simulink model "State_feedback_controller"  (R2020a)
settings: Solver=VariableStepAuto  StartTime=0.0  StopTime=10.0  RelTol=1e-3
undefined symbols (not defined in the file): Ad, bd, c, d, K1, K2, T
settings Model: Creator=elkin  LastModifiedBy=elkin

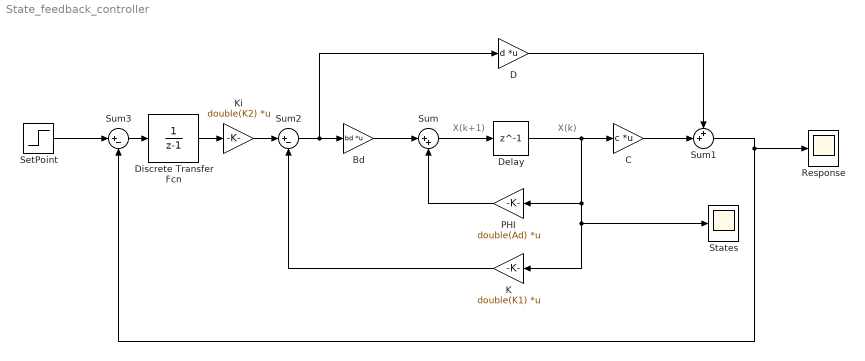
== system State_feedback_controller ==
  note: X(k+1)
  note: X(k)
  Bd : Gain  Gain=bd  Multiplication=Matrix(K*u)
  C : Gain  Gain=c  Multiplication=Matrix(K*u)
  D : Gain  Gain=d  Multiplication=Matrix(K*u)
  Delay : Delay  DelayLength=1  SampleTime=T
  Discrete Transfer Fcn : DiscreteTransferFcn  Denominator=[1 -1]  SampleTime=T
  K : Gain  Gain=double(K1)  Multiplication=Matrix(K*u)
  Ki : Gain  Gain=double(K2)  Multiplication=Matrix(K*u)
  PHI : Gain  Gain=double(Ad)  Multiplication=Matrix(K*u)
  Response : Scope
  SetPoint : Step  Time=0  SampleTime=0
  States : Scope
  Sum : Sum  Inputs=|++
  Sum1 : Sum  Inputs=++|
  Sum2 : Sum  Inputs=|+-
  Sum3 : Sum  Inputs=|+-
  wires:
  Bd/1 -> Sum/1
  Sum/1 -> Delay/1
  PHI/1 -> Sum/2
  Delay/1 -> States/1, K/1, PHI/1, C/1
  D/1 -> Sum1/1
  C/1 -> Sum1/2
  Sum1/1 -> Sum3/2, Response/1
  Sum2/1 -> D/1, Bd/1
  K/1 -> Sum2/2
  SetPoint/1 -> Sum3/1
  Ki/1 -> Sum2/1
  Discrete Transfer Fcn/1 -> Ki/1
  Sum3/1 -> Discrete Transfer Fcn/1
